simulink model "sampleModel1537"  (R2023a)
settings: Solver=VariableStepAuto  StartTime=0.0  StopTime=10.0  RelTol=1e-3
libraries: simulink x3, hdlsllib x1
settings Model: Creator=user1  LastModifiedBy=user1

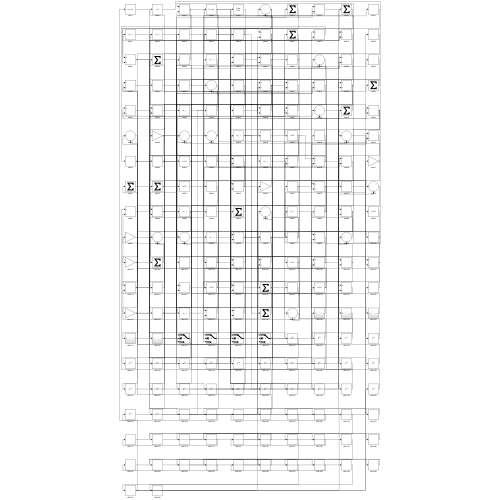
[thumbnail: Simulink's stored preview of the top-level diagram]
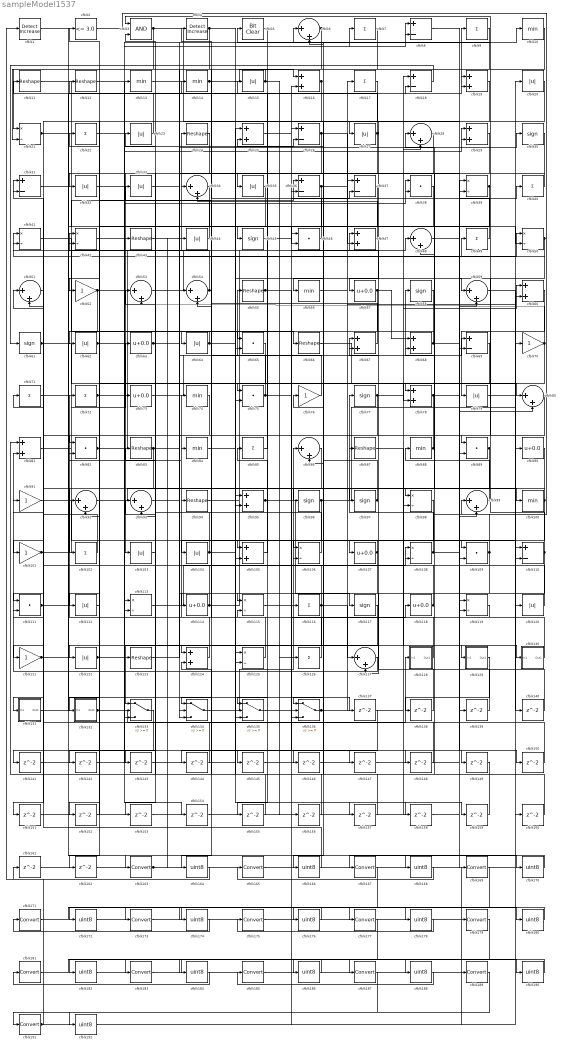
== system sampleModel1537 ==
  cfblk1 : simulink/Logic and Bit Operations/Detect Increase  vinit=0.0  OutDataTypeStr=boolean
      settings: LibrarySourceBlock=|
      | hdlsllib/Logic and Bit
      | Operations/Detect
      | Increase
  cfblk{10,13..14,56,74,84,88,100} (8 alike) : MinMax
  cfblk{52,70,76,91,101,121} (6 alike) : Gain
  cfblk{7,9,17,22,40,49,71..72,85,102,116,126} (12 alike) : Sum  Inputs=+
  cfblk{15,20,23,27,32..33,35,44,62,64,79,103..104,112,120,122} (16 alike) : Abs  SaturateOnIntegerOverflow=off
  cfblk{16,19,25,29,47,60,67..68,78,81,95,105,124} (13 alike) : Sum
  cfblk{21,39,41..42,50,98,106,108,113,115,119,125} (12 alike) : Product  Inputs=*/  RndMeth=Zero  SaturateOnIntegerOverflow=on
  cfblk{57,63,73,90,107,114,118} (7 alike) : Bias  Bias=0.0  SaturateOnIntegerOverflow=off
  cfblk{38,46,65,75,82,89,109,111} (8 alike) : DotProduct  OutDataTypeStr=Inherit: Inherit via internal rule
  cfblk{11..12,24,43,55,66,83,87,94,123} (10 alike) : Reshape
  cfblk{8,18,26,31,36..37,69,110} (8 alike) : Sum  Inputs=+-
  cfblk{30,45,58,61,77,96..97,117} (8 alike) : Signum
  cfblk{6,28,34,48,51,53..54,59,80,86,92..93,99,127} (14 alike) : Sum  Inputs=|++
  cfblk128 : Subsystem
      settings: LibrarySourceBlock=|
      | hdlsllib/Ports &
      | Subsystems/Subsystem
  cfblk129 : Subsystem
      settings: LibrarySourceBlock=|
      | hdlsllib/Ports &
      | Subsystems/Subsystem
  cfblk130 : Subsystem
      settings: LibrarySourceBlock=|
      | hdlsllib/Ports &
      | Subsystems/Subsystem
  cfblk131 : Subsystem
      settings: LibrarySourceBlock=|
      | hdlsllib/Ports &
      | Subsystems/Subsystem
  cfblk132 : Subsystem
      settings: LibrarySourceBlock=|
      | hdlsllib/Ports &
      | Subsystems/Subsystem
  cfblk{133..136} (4 alike) : Switch  SaturateOnIntegerOverflow=off  InputSameDT=off
  cfblk{137..162} (26 alike) : Delay  SampleTime=1
  cfblk{163,165,167,169,171,173,175,177,179,181,183,185,187,189,191} (15 alike) : DataTypeConversion  SaturateOnIntegerOverflow=off  RndMeth=Floor
  cfblk{164,166,168,170,172,174,176,178,180,182,184,186,188,190,192} (15 alike) : DataTypeConversion  OutDataTypeStr=uint8  SaturateOnIntegerOverflow=off  RndMeth=Floor
  cfblk2 : hdlsllib/Logic and Bit Operations/Compare To Constant  relop=<=  const=3.0  OutDataTypeStr=boolean
  cfblk3 : Logic  AllPortsSameDT=off  OutDataTypeStr=boolean
  cfblk4 : simulink/Logic and Bit Operations/Detect Increase  vinit=0.0  OutDataTypeStr=boolean
      settings: LibrarySourceBlock=|
      | hdlsllib/Logic and Bit
      | Operations/Detect
      | Increase
  cfblk5 : simulink/Logic and Bit Operations/Bit Clear  iBit=0
      settings: LibrarySourceBlock=|
      | hdlsllib/Logic and Bit
      | Operations/Bit Clear
  wires:
  cfblk26/1 -> cfblk103/1, cfblk50/2
  cfblk11/1 -> cfblk43/1
  cfblk74/1 -> cfblk122/1
  cfblk15/1 -> cfblk21/1, cfblk156/1
  cfblk97/1 -> cfblk77/1, cfblk25/2
  cfblk36/1 -> cfblk29/1, cfblk135/3, cfblk142/1
  cfblk13/1 -> cfblk9/1
  cfblk95/1 -> cfblk117/1, cfblk109/1
  cfblk75/1 -> cfblk54/2, cfblk149/1
  cfblk94/1 -> cfblk100/1
  cfblk115/1 -> cfblk86/1
  cfblk60/1 -> cfblk79/1
  cfblk127/1 -> cfblk81/2
  cfblk39/1 -> cfblk3/1, cfblk52/1, cfblk65/2
  cfblk81/1 -> cfblk36/1
  cfblk92/1 -> cfblk96/1
  cfblk114/1 -> cfblk47/1, cfblk31/2
  cfblk61/1 -> cfblk80/1, cfblk147/1
  cfblk64/1 -> cfblk62/1, cfblk158/1
  cfblk2/1 -> cfblk99/1
  cfblk102/1 -> cfblk31/1
  cfblk107/1 -> cfblk106/1, cfblk134/3
  cfblk30/1 -> cfblk32/1
  cfblk76/1 -> cfblk55/1
  cfblk96/1 -> cfblk70/1, cfblk60/1, cfblk135/2
  cfblk18/1 -> cfblk61/1
  cfblk82/1 -> cfblk24/1, cfblk130/1(In1)
  cfblk122/1 -> cfblk13/1, cfblk38/2
  cfblk126/1 -> cfblk72/1
  cfblk3/1 -> cfblk119/1, cfblk42/2
  cfblk101/1 -> cfblk63/1, cfblk151/1
  cfblk66/1 -> cfblk110/1
  cfblk6/1 -> cfblk124/1, cfblk105/2
  cfblk27/1 -> cfblk11/1, cfblk73/1
  cfblk58/1 -> cfblk136/1
  cfblk134/1 -> cfblk106/2
  cfblk12/1 -> cfblk107/1
  cfblk70/1 -> cfblk132/1(In1), cfblk53/2
  cfblk105/1 -> cfblk85/1
  cfblk19/1 -> cfblk112/1
  cfblk41/1 -> cfblk64/1
  cfblk4/1 -> cfblk59/1, cfblk134/2, cfblk137/1
  cfblk16/1 -> cfblk111/1, cfblk45/1
  cfblk83/1 -> cfblk102/1, cfblk50/1, cfblk7/1
  cfblk9/1 -> cfblk21/2
  cfblk49/1 -> cfblk14/1
  cfblk63/1 -> cfblk8/1, cfblk78/2
  cfblk73/1 -> cfblk58/1
  cfblk1/1 -> cfblk163/1
  cfblk128/1(Out1) -> cfblk76/1
  cfblk109/1 -> cfblk28/1, cfblk114/1
  cfblk59/1 -> cfblk90/1
  cfblk44/1 -> cfblk22/1
  cfblk72/1 -> cfblk12/1, cfblk154/1
  cfblk78/1 -> cfblk80/2, cfblk145/1
  cfblk67/1 -> cfblk33/1
  cfblk50/1 -> cfblk89/1, cfblk41/2, cfblk89/2
  cfblk35/1 -> cfblk125/2
  cfblk46/1 -> cfblk4/1
  cfblk135/1 -> cfblk118/1
  cfblk21/1 -> cfblk136/2, cfblk148/1
  cfblk106/1 -> cfblk53/1
  cfblk53/1 -> cfblk37/1
  cfblk136/1 -> cfblk17/1, cfblk18/1
  cfblk91/1 -> cfblk105/1
  cfblk118/1 -> cfblk74/1, cfblk68/2
  cfblk99/1 -> cfblk88/1
  cfblk45/1 -> cfblk36/2
  cfblk40/1 -> cfblk35/1
  cfblk28/1 -> cfblk56/1
  cfblk130/1(Out1) -> cfblk34/1
  cfblk32/1 -> cfblk26/2
  cfblk10/1 -> cfblk115/1
  cfblk125/1 -> cfblk93/1
  cfblk52/1 -> cfblk110/2, cfblk10/1, cfblk82/2
  cfblk131/1(Out1) -> cfblk48/1
  cfblk117/1 -> cfblk133/1
  cfblk112/1 -> cfblk42/1
  cfblk119/1 -> cfblk115/2
  cfblk43/1 -> cfblk30/1
  cfblk120/1 -> cfblk6/1
  cfblk132/1(Out1) -> cfblk128/1(In1), cfblk29/2
  cfblk47/1 -> cfblk34/2
  cfblk84/1 -> cfblk67/1
  cfblk55/1 -> cfblk116/1, cfblk126/1, cfblk37/2
  cfblk42/1 -> cfblk66/1
  cfblk90/1 -> cfblk121/1
  cfblk77/1 -> cfblk131/1(In1), cfblk60/2
  cfblk25/1 -> cfblk27/1
  cfblk116/1 -> cfblk127/1, cfblk51/2, cfblk152/1
  cfblk103/1 -> cfblk83/1
  cfblk108/1 -> cfblk87/1, cfblk40/1
  cfblk34/1 -> cfblk133/2
  cfblk14/1 -> cfblk16/1, cfblk157/1
  cfblk104/1 -> cfblk41/1, cfblk159/1
  cfblk62/1 -> cfblk19/1, cfblk38/1, cfblk8/2
  cfblk110/1 -> cfblk5/1, cfblk127/2
  cfblk23/1 -> cfblk2/1
  cfblk113/1 -> cfblk108/1
  cfblk124/1 -> cfblk94/1
  cfblk20/1 -> cfblk57/1
  cfblk111/1 -> cfblk92/1, cfblk19/2, cfblk91/1
  cfblk85/1 -> cfblk15/1
  cfblk31/1 -> cfblk47/2
  cfblk80/1 -> cfblk123/1
  cfblk57/1 -> cfblk133/3, cfblk68/1, cfblk162/1
  cfblk88/1 -> cfblk48/2, cfblk82/1
  cfblk65/1 -> cfblk75/1
  cfblk7/1 -> cfblk104/1
  cfblk86/1 -> cfblk113/2
  cfblk51/1 -> cfblk101/1
  cfblk123/1 -> cfblk54/1
  cfblk87/1 -> cfblk129/1(In1)
  cfblk29/1 -> cfblk78/1
  cfblk68/1 -> cfblk99/2, cfblk65/1
  cfblk56/1 -> cfblk49/1
  cfblk121/1 -> cfblk84/1, cfblk18/2
  cfblk54/1 -> cfblk23/1, cfblk144/1
  cfblk69/1 -> cfblk98/1
  cfblk38/1 -> cfblk75/2
  cfblk93/1 -> cfblk69/1
  cfblk89/1 -> cfblk95/2, cfblk135/1
  cfblk100/1 -> cfblk97/1, cfblk134/1
  cfblk22/1 -> cfblk46/2
  cfblk33/1 -> cfblk39/2
  cfblk129/1(Out1) -> cfblk138/1
  cfblk138/1 -> cfblk46/1
  cfblk48/1 -> cfblk139/1
  cfblk139/1 -> cfblk67/2
  cfblk79/1 -> cfblk140/1
  cfblk140/1 -> cfblk39/1
  cfblk133/1 -> cfblk141/1
  cfblk141/1 -> cfblk113/1
  cfblk142/1 -> cfblk125/1
  cfblk24/1 -> cfblk143/1
  cfblk143/1 -> cfblk95/1
  cfblk144/1 -> cfblk3/2
  cfblk145/1 -> cfblk69/2
  cfblk17/1 -> cfblk146/1
  cfblk146/1 -> cfblk86/2
  cfblk147/1 -> cfblk98/2
  cfblk148/1 -> cfblk111/2
  cfblk149/1 -> cfblk81/1
  cfblk8/1 -> cfblk150/1
  cfblk150/1 -> cfblk51/1
  cfblk151/1 -> cfblk28/2
  cfblk152/1 -> cfblk92/2
  cfblk37/1 -> cfblk153/1
  cfblk153/1 -> cfblk26/1
  cfblk154/1 -> cfblk109/2
  cfblk5/1 -> cfblk155/1
  cfblk155/1 -> cfblk124/2
  cfblk156/1 -> cfblk25/1
  cfblk157/1 -> cfblk6/2
  cfblk158/1 -> cfblk59/2
  cfblk159/1 -> cfblk93/2
  cfblk160/1 -> cfblk108/2
  cfblk161/1 -> cfblk119/2
  cfblk162/1 -> cfblk20/1
  cfblk163/1 -> cfblk136/3, cfblk44/1
  cfblk137/1 -> cfblk164/1
  cfblk164/1 -> cfblk1/1
  cfblk98/1 -> cfblk166/1
  cfblk166/1 -> cfblk71/1
  cfblk71/1 -> cfblk168/1
  cfblk168/1 -> cfblk165/1
  cfblk165/1 -> cfblk170/1
  cfblk170/1 -> cfblk167/1
  cfblk167/1 -> cfblk172/1
  cfblk172/1 -> cfblk169/1
  cfblk169/1 -> cfblk174/1
  cfblk174/1 -> cfblk171/1
  cfblk171/1 -> cfblk176/1
  cfblk176/1 -> cfblk173/1
  cfblk173/1 -> cfblk178/1
  cfblk178/1 -> cfblk175/1
  cfblk175/1 -> cfblk180/1
  cfblk180/1 -> cfblk177/1
  cfblk177/1 -> cfblk182/1
  cfblk182/1 -> cfblk179/1
  cfblk179/1 -> cfblk184/1
  cfblk184/1 -> cfblk181/1
  cfblk181/1 -> cfblk186/1
  cfblk186/1 -> cfblk183/1
  cfblk183/1 -> cfblk188/1
  cfblk188/1 -> cfblk185/1
  cfblk189/1 -> cfblk191/1
  cfblk185/1 -> cfblk190/1
  cfblk190/1 -> cfblk187/1
  cfblk191/1 -> cfblk120/1, cfblk16/2, cfblk160/1, cfblk161/1
  cfblk187/1 -> cfblk192/1
  cfblk192/1 -> cfblk189/1

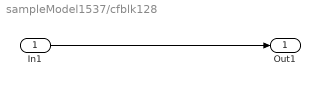
== system sampleModel1537/cfblk128 ==
  In1 : Inport
  Out1 : Outport
  wires:
  In1/1 -> Out1/1

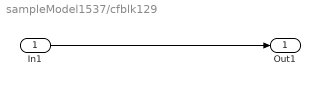
== system sampleModel1537/cfblk129 ==
  In1 : Inport
  Out1 : Outport
  wires:
  In1/1 -> Out1/1

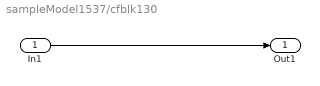
== system sampleModel1537/cfblk130 ==
  In1 : Inport
  Out1 : Outport
  wires:
  In1/1 -> Out1/1

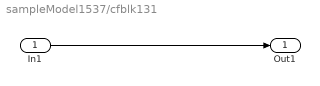
== system sampleModel1537/cfblk131 ==
  In1 : Inport
  Out1 : Outport
  wires:
  In1/1 -> Out1/1

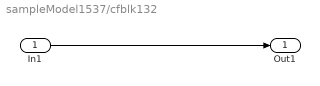
== system sampleModel1537/cfblk132 ==
  In1 : Inport
  Out1 : Outport
  wires:
  In1/1 -> Out1/1
